simulink model "test_beam"  (R2020b)
settings: Solver=VariableStepAuto  StartTime=0.0  StopTime=10.0  RelTol=1e-3
undefined symbols (not defined in the file): const, mech
settings Model: Creator=Utente  LastModifiedBy=Utente

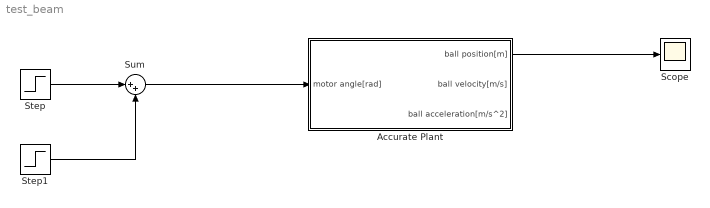
== system test_beam ==
  Accurate Plant : Subsystem
  Scope : Scope
  Step : Step  Time=0  After=-pi/180  SampleTime=0
  Step1 : Step  Time=2.5  After=2*pi/180  SampleTime=0
  Sum : Sum  Inputs=|++
  wires:
  Accurate Plant/1(ball position[m]) -> Scope/1
  Step/1 -> Sum/1
  Step1/1 -> Sum/2
  Sum/1 -> Accurate Plant/1(motor angle[rad])

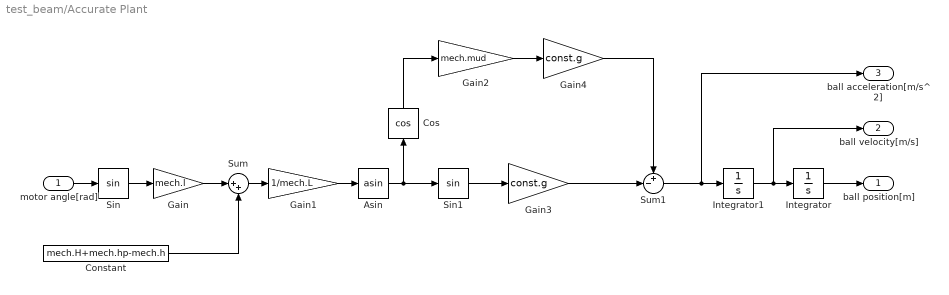
== system test_beam/Accurate Plant ==
  motor angle[rad] : Inport
  Asin : Trigonometry  Operator=asin
  Constant : Constant  Value=mech.H+mech.hp-mech.h
  Cos : Trigonometry  Operator=cos
  Gain : Gain  Gain=mech.l
  Gain1 : Gain  Gain=1/mech.L
  Gain2 : Gain  Gain=mech.mud
  Gain3 : Gain  Gain=const.g
  Gain4 : Gain  Gain=const.g
  Integrator : Integrator
  Integrator1 : Integrator
  Sin : Trigonometry
  Sin1 : Trigonometry
  Sum : Sum  Inputs=|++
  Sum1 : Sum  Inputs=+-|
  ball position[m] : Outport
  ball velocity[m/s] : Outport  Port=2
  ball acceleration[m/s^2] : Outport  Port=3
  wires:
  Integrator/1 -> ball position[m]/1
  Integrator1/1 -> ball velocity[m/s]/1, Integrator/1
  Sum1/1 -> ball acceleration[m/s^2]/1, Integrator1/1
  motor angle[rad]/1 -> Sin/1
  Sin/1 -> Gain/1
  Gain/1 -> Sum/1
  Constant/1 -> Sum/2
  Gain1/1 -> Asin/1
  Sum/1 -> Gain1/1
  Asin/1 -> Sin1/1, Cos/1
  Sin1/1 -> Gain3/1
  Gain3/1 -> Sum1/2
  Cos/1 -> Gain2/1
  Gain2/1 -> Gain4/1
  Gain4/1 -> Sum1/1
